simulink model "Test_model"  (R2021a)
settings: Solver=VariableStepAuto  StartTime=0.0  StopTime=1  RelTol=1e-3
undefined symbols (not defined in the file or in its folder): ADMM_struct, constraints_struct, model, Objective
settings Model: Creator=worc4873  LastModifiedBy=worc4873

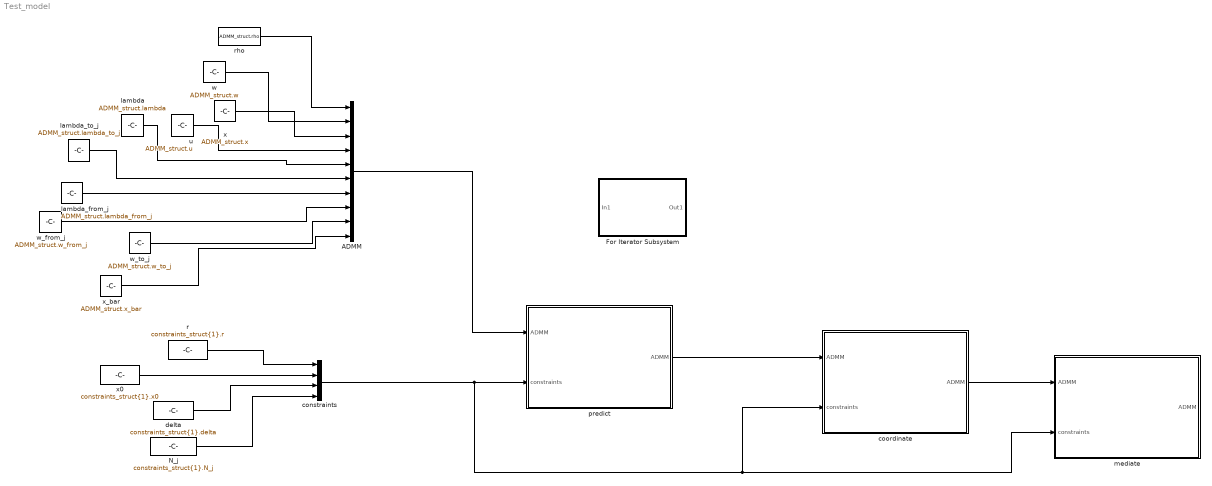
== system Test_model ==
  ADMM : BusCreator  Inputs=10
  For Iterator Subsystem : Subsystem  TreatAsAtomicUnit=on
  N_j : Constant  Value=constraints_struct{1}.N_j
  constraints : BusCreator  Inputs=4
  coordinate : MATLAB Function  TreatAsAtomicUnit=on
  delta : Constant  Value=constraints_struct{1}.delta
  lambda : Constant  Value=ADMM_struct.lambda
  lambda_from_j : Constant  Value=ADMM_struct.lambda_from_j
  lambda_to_j : Constant  Value=ADMM_struct.lambda_to_j
  mediate : MATLAB Function  TreatAsAtomicUnit=on
  predict : MATLAB Function  TreatAsAtomicUnit=on
  r : Constant  Value=constraints_struct{1}.r
  rho : Constant  Value=ADMM_struct.rho
  u : Constant  Value=ADMM_struct.u
  w : Constant  Value=ADMM_struct.w
  w_from_j : Constant  Value=ADMM_struct.w_from_j
  w_to_j : Constant  Value=ADMM_struct.w_to_j
  x : Constant  Value=ADMM_struct.x
  x0 : Constant  Value=constraints_struct{1}.x0
  x_bar : Constant  Value=ADMM_struct.x_bar
  wires:
  ADMM/1 -> predict/1("ADMM ")
  N_j/1 -> constraints/4
  r/1 -> constraints/1
  x0/1 -> constraints/2
  predict/1(ADMM) -> coordinate/1("ADMM ")
  coordinate/1(ADMM) -> mediate/1("ADMM ")
  rho/1 -> ADMM/1
  w/1 -> ADMM/2
  x/1 -> ADMM/3
  lambda/1 -> ADMM/5
  lambda_to_j/1 -> ADMM/6
  lambda_from_j/1 -> ADMM/7
  w_from_j/1 -> ADMM/8
  w_to_j/1 -> ADMM/9
  x_bar/1 -> ADMM/10
  u/1 -> ADMM/4
  constraints/1 -> mediate/2(constraints), coordinate/2(constraints), predict/2(constraints)
  delta/1 -> constraints/3

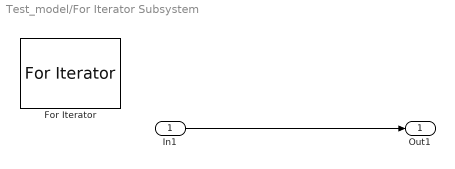
== system Test_model/For Iterator Subsystem ==
  In1 : Inport
  For Iterator : ForIterator
  Out1 : Outport
  wires:
  In1/1 -> Out1/1

== matlab function Test_model/coordinate ==
  data: ADMM input Bus: ADMM; ADMM output; Objective parameter; constraints input Bus: constraints
function ADMM = coordinate_step(ADMM,Objective, constraints)

Nd = 3;
nx = size(Objective.Q,1);
nu = size(Objective.R,1);

N = Objective.N;

d = [eye(Nd),zeros(Nd,nx-Nd)]; % Matrix to take only position from the state vector x (only returns pos)
posMN = kron(eye(N+1),d); %returns pos across time steps


rhoM = kron(speye((N+1)),ADMM.rho/2*eye(nu)); % matrix for the quadratic objective formualation
Pc = kron(eye(1+size(constraints.N_j,2)),rhoM);

H = kron(eye(N+1),repmat(d, size(constraints.N_j,2), 1));
Hw = kron(eye(N+1),repmat(eye(nu), size(constraints.N_j,2), 1));
for j = 1:size(constraints.N_j,2)
    v = zeros(size(constraints.N_j,2),1);
    v(j) = 1;
    H_M = kron(eye(N+1),kron(v, -1*d));
    H_Mw = kron(eye(N+1),kron(v, -1*eye(nu)));
    
    H =  [H, H_M];
    Hw = [Hw,H_Mw];
end
qc = coordination_linear(ADMM.lambda,ADMM.lambda_to_j,ADMM.rho,ADMM.x_bar,posMN);

% Update matrices

qp_opts = optimoptions('quadprog','Display','off','Algorithm','active-set');
init = ADMM.w;
for j = 1:size(constraints.N_j,2)
   init = [init;ADMM.w_to_j(:,j)]; 
end
[A_ineq,l_ineq] = communicate(ADMM.x_bar,Objective.N,constraints.N_j,H,Hw,constraints.delta,nu);
resc = quadprog(full(Pc),qc,-A_ineq,-l_ineq,[],[],[],[],init,qp_opts);


ADMM.w = resc(1:Nd*(N+1),1);
for j = 1:size(constraints.N_j,2)
    ADMM.w_to_j(:,j) = resc(j*Nd*(N+1)+1:(j+1)*Nd*(N+1),1);
end

end

== matlab function Test_model/predict ==
  data: ADMM input Bus: ADMM; ADMM output; Objective parameter; model parameter; constraints input Bus: constraints
function ADMM = predict_step(ADMM,Objective, model, constraints)

Q = Objective.Q;
R = Objective.R;
N = Objective.N;

Nd = 3;
nx = size(Q,1);
nu = size(R,1);

A = model.A;
B = model.B;
umax = model.umax;
umin = model.umin;


N_j = constraints.N_j;
r = constraints.r;
x0 = constraints.x0;

rho = ADMM.rho;
lambda = ADMM.lambda;
lambda_from_j = ADMM.lambda_from_j;
w = ADMM.w;
w_from_j = ADMM.w_from_j;

min_input = repmat(ones(nu,1)*umin,N,1);
max_input = repmat(ones(nu,1)*umax,N,1);
% - linear dynamics

u_bound = [inf((N+1)*nx,1);max_input];
l_bound = [-inf((N+1)*nx,1);min_input];


posM = blkdiag(eye(Nd),zeros(nx-Nd)); % Matrix to take only position from the state vector x (zeros rest)
d = [eye(Nd),zeros(Nd,nx-Nd)]; % Matrix to take only position from the state vector x (only returns pos)
posMN = kron(eye(N+1),d); %returns pos across time steps

Ax = kron(speye(N+1), -speye(nx)) + kron(sparse(diag(ones(N, 1), -1)), A);
Bu = kron([sparse(1, N); speye(N)], B);
Aeq = [Ax, Bu];
b_eq = [-x0'; zeros(N*nx, 1)];
P_new = blkdiag( kron(eye(N), Q+ (size(N_j,2)+1)*rho/2*posM ), Q+(size(N_j,2)+1)*rho/2*posM, kron(eye(N), R) );

q = prediction_linear(lambda,lambda_from_j,w,w_from_j,rho,r',Q,N,nu,posMN);

qp_opts = optimoptions('quadprog','Display','off','Algorithm','active-set');
init = [ADMM.x;ADMM.u];
res = quadprog(P_new,q,[],[], full(Aeq),b_eq,l_bound,u_bound,init,qp_opts);
ADMM.x = res(1:nx*(N+1));
ADMM.u = res((N+1)*nx+1:end);

end

== matlab function Test_model/mediate ==
  data: ADMM input Bus: ADMM; ADMM output; N parameter; constraints input Bus: constraints
function ADMM = mediate_step(ADMM,N, constraints)

Nd = 3;
nx = size(ADMM.x,1)/(N+1);

d = [eye(Nd),zeros(Nd,nx-Nd)]; % Matrix to take only position from the state vector x (only returns pos)
posMN = kron(eye(N+1),d); %returns pos across time steps


ADMM.lambda = ADMM.lambda + ADMM.rho * (posMN * ADMM.x-ADMM.w);
for j = 1:size(constraints.N_j,2)
    ADMM.lambda_to_j(:,j) = ADMM.lambda_to_j(:,j) + ADMM.rho * (posMN*ADMM.x_bar(:,j+1) - ADMM.w_to_j(:,j));
end

end
